simulink model "New_saturationvalue_water"  (Simulink 7.9)
settings: Solver=FixedStepDiscrete  StartTime=0.0  StopTime=10  FixedStep=1  RelTol=1e-3
undefined symbols (not defined in the file): Carnot_saturationvalue_water_Callbacks
settings Model: Creator=awohlfei  LastModifiedBy=awohlfei

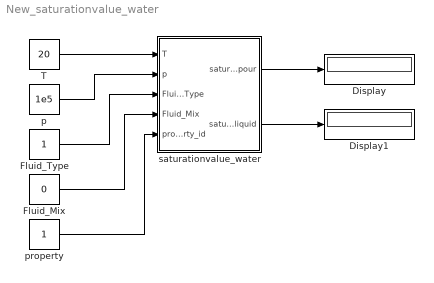
== system New_saturationvalue_water ==
  Display : Display
  Display1 : Display
  Fluid_Mix : Constant  Value=0
  Fluid_Type : Constant
  T : Constant  Value=20
  p : Constant  Value=1e5
  property : Constant
  saturationvalue_water : Subsystem  LoadFcn=Carnot_saturationvalue_water_Callbacks('LoadFcn');  InitFcn=load('THB.mat');  VariantObject=CarlibClassic  mask(saturation value water){INPUTARGUMENTS=state variables (classic), DEBUGLEVEL=WARNING, MAXTOTALMESSAGES=inf, MAXCONSECUTIVEMESSAGES=inf, WRITETOFILE=0, FILENAME='errors.txt'}
      mask prompts: INPUTARGUMENTS "Input arguments"; DEBUGLEVEL "Debug level"; MAXTOTALMESSAGES "maximum number of total warning"; MAXCONSECUTIVEMESSAGES "maximum number of consecutive warnings"; WRITETOFILE "write messages to file"; FILENAME "filename for error messages"
      mask help:
      | The block calculates the saturation value of fluid
      | by the value of a specified property.
      | Calls the function "saturationproperty" in the CARNOT library "Carlib".
      |
      | Definition of property-types
      | property-ID        property                       unit
      | 1                       density                         [kg/m³]
      | 2                       heat capacity               [J/kgK]
      | 3                       heat conductivity         [W/mK]
      | 4                       kinematic viscosity       [m²/s]
      | 5                       enthalpy                       [J/kg]
      | 6                       entropy                         [J/kgK]
      | 7                       prandtl                          [-]
      | 8                       specific volume            [m³/kg]
      |
      | not defined for this function
      | 9                       evaporation  enthalpy  [J/kg]
      | 10                     vapourpressure            [Pa]
      | 11                     saturationtemperatur    [°C]
      mask init:
      | %Inports
      | Carnot_saturationvalue_water_Callbacks('CreateInports');
      | 
      | %global debug level
      | [DEBUGLEVEL, MAXTOTALMESSAGES, MAXCONSECUTIVEMESSAGES, WRITETOFILE, FILENAME] = Carnot_saturationvalue_water_Callbacks('CheckDebugLevels', DEBUGLEVEL, MAXTOTALMESSAGES, MAXCONSECUTIVEMESSAGES, WRITETOFILE, FILENAME);
      mask Help: eval('man(''saturationvalue_water'')')
      mask StyleString: popup(state variables (classic)|THB|THV),popup(DEBUG|INFO|WARNING|ERROR|FATAL|NONE),edit,edit,edit,edit
      mask CallbackString: Carnot_saturationvalue_water_Callbacks('MaskVisibilities');|||||
      mask TabNameString: Parameters,Debugging,Debugging,Debugging,Debugging,Debugging
  wires:
  saturationvalue_water/1(saturation_vapour) -> Display/1
  T/1 -> saturationvalue_water/1(T)
  p/1 -> saturationvalue_water/2(p)
  Fluid_Type/1 -> saturationvalue_water/3(Fluid_Type)
  Fluid_Mix/1 -> saturationvalue_water/4(Fluid_Mix)
  property/1 -> saturationvalue_water/5(property_id)
  saturationvalue_water/2(saturation_liquid) -> Display1/1

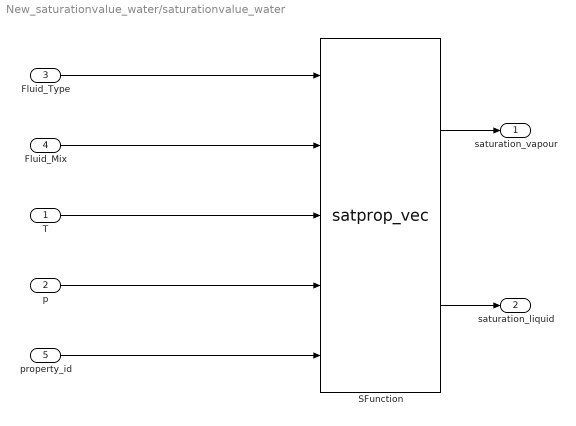
== system New_saturationvalue_water/saturationvalue_water ==
  T : Inport
  p : Inport  Port=2
  Fluid_Type : Inport  Port=3
  Fluid_Mix : Inport  Port=4
  property_id : Inport  Port=5
  SFunction : S-Function  FunctionName=satprop_vec  Parameters=DEBUGLEVEL,MAXTOTALMESSAGES,MAXCONSECUTIVEMESSAGES,WRITETOFILE,FILENAME  EnableBusSupport=off
  saturation_vapour : Outport
  saturation_liquid : Outport  Port=2
  wires:
  SFunction/1 -> saturation_vapour/1
  SFunction/2 -> saturation_liquid/1
  T/1 -> SFunction/3
  p/1 -> SFunction/4
  Fluid_Type/1 -> SFunction/1
  Fluid_Mix/1 -> SFunction/2
  property_id/1 -> SFunction/5
